simulink model "flare_mode"  (R2020b)
settings: Solver=VariableStepAuto  StartTime=0.0  StopTime=10.0  RelTol=1e-3
values from neighbouring files (symbols this model uses):
  Initial_elevator = -4.1    [Masterscript.m]
  Initial_throttle = 1000    [Masterscript.m]
  tau = 1.1233    [Masterscript.m]
  V_ref = 300    [Masterscript.m]
libraries: pid_lib x4, dspmathops x2
settings Model: Creator=niekv  LastModifiedBy=niekv

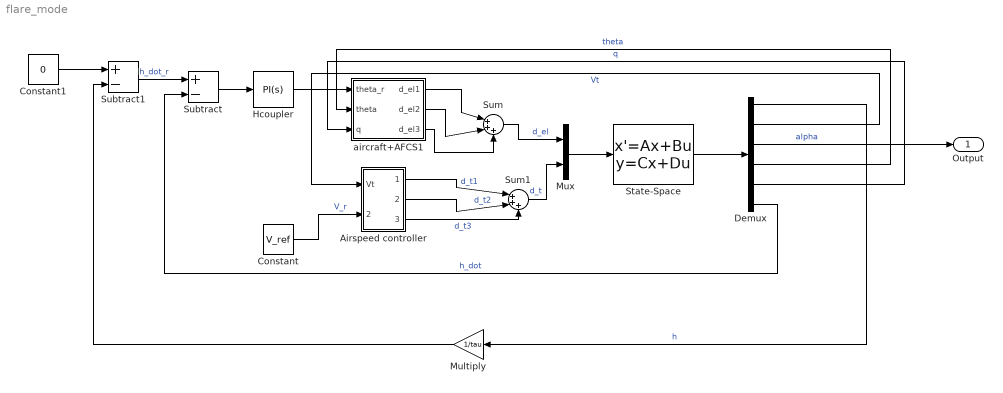
== system flare_mode ==
  Airspeed controller : Subsystem
  Constant : Constant  Value=V_ref
  Constant1 : Constant  Value=0
  Demux : Demux  Outputs=6
  Hcoupler : pid_lib/PID Controller  Controller=PI  Form=Parallel  TimeDomain=Continuous-time  UseExternalTs=off  SampleTime=-1  IntegratorMethod=Forward Euler  FilterMethod=Forward Euler  ControllerParametersSource=internal  P=1  I=0.1  D=0  UseFilter=on  N=100  TunerSelectOption=Transfer Function Based (PID Tuner App)  InitialConditionSource=internal  InitialConditionForIntegrator=0  InitialConditionForFilter=0  DifferentiatorICPrevScaledInput=0  ExternalReset=none  TrackingMode=off  Kt=1  LimitOutput=off  SatLimitsSource=internal  UpperSaturationLimit=inf  LowerSaturationLimit=-inf  LinearizeAsGain=on  AntiWindupMode=none  Kb=1  POutMin=[]  POutMax=[]  IOutMin=[]  IOutMax=[]  DOutMin=[]  DOutMax=[]  NOutMin=[]  NOutMax=[]  SumOutMin=[]  SumOutMax=[]  SaturationOutMin=[]  SaturationOutMax=[]  PParamMin=[]  PParamMax=[]  IParamMin=[]  IParamMax=[]  DParamMin=[]  DParamMax=[]  NParamMin=[]  NParamMax=[]  KbParamMin=[]  KbParamMax=[]  KtParamMin=[]  KtParamMax=[]  KbOutMin=[]  KbOutMax=[]  KtOutMin=[]  KtOutMax=[]  IntegratorOutMin=[]  IntegratorOutMax=[]  FilterOutMin=[]  FilterOutMax=[]  SumI1OutMin=[]  SumI1OutMax=[]  SumI2OutMin=[]  SumI2OutMax=[]  SumI3OutMin=[]  SumI3OutMax=[]  SumI4OutMin=[]  SumI4OutMax=[]  SumDOutMin=[]  SumDOutMax=[]  DifferentiatorOutMin=[]  DifferentiatorOutMax=[]  FilterDiffOutCoefMin=[]  FilterDiffOutCoefMax=[]  ReciprocalOutMin=[]  ReciprocalOutMax=[]  SumDenOutMin=[]  SumDenOutMax=[]  SumNumOutMin=[]  SumNumOutMax=[]  DivideOutMin=[]  DivideOutMax=[]  UdiffTsProdOutMin=[]  UdiffTsProdOutMax=[]  NTsProdOutMin=[]  NTsProdOutMax=[]  UintegralTsProdOutMin=[]  UintegralTsProdOutMax=[]  UngainTsProdOutMin=[]  UngainTsProdOutMax=[]  IntegratorContinuousStateAttributes=''  IntegratorStateMustResolveToSignalObject=off  IntegratorRTWStateStorageClass=Auto  FilterContinuousStateAttributes=''  FilterStateMustResolveToSignalObject=off  FilterRTWStateStorageClass=Auto  ParallelPVariant=InternalParameters  IdealPVariant=Disabled  IVariant=InternalParameters  DVariant=Disabled  IntegratorVariant=Continuous  SatVariant=Disabled  AWVariant=Passthrough  PCopyVariant=Disabled  TRVariant=Disabled  FdbkBlocksVariant=Forward  IdealPFdbkVariant=Disabled  SatFdbkVariant=Disabled  DerivativeFilterVariant=Disabled  NVariant=Disabled  NCopyVariant=Disabled_SignalSpec  FilterICVariant=Disabled  IntegratorICVariant=InternalICs  ExternalResetVariant=Disabled  TRSumVariant=Passthrough  SumFdbkVariant=Disabled  SumVariant=Sum_PI  TsampFilterVariant=InternalTs  TsampNgainVariant=Passthrough  TsampIntegralVariant=Passthrough  ExternalSaturationOutDataTypeStr=Inherit: Same as second input
  Multiply : Gain  Gain=1/tau
  Mux : Mux  Inputs=2
  State-Space : StateSpace  A=[0 0 -300 300 0; 0.0001317 -0.0291 2.13 -32.17 -2.895; 3.154e-06 -0.000697 -0.5447 4.55e-13 0.9152; 0 0 0 0 1; -4.699e-21 1.038e-18 0.3303 0 -0.8169]  B=[0 0; -0.004534 0.001544; -0.001116 -9.493e-07; 0 0 ; -0.05702 0]  C=[1 0 0 0 0; 0 1 0 0 0; 0 0 1 0 0; 0 0 0 1 0; 0 0 0 0 1; 0 0 -300 300 0]  D=[0 0; 0 0; 0 0; 0 0; 0 0; 0 0]  InitialCondition=[5000; 300; 10.4511; 10.4511; 0]  ContinuousStateAttributes={'h', 'Vt', 'alpha', 'theta', 'q'}
  Subtract : Sum  Inputs=+-
  Subtract1 : Sum  Inputs=+-
  Sum : Sum  Inputs=|+++
  Sum1 : Sum  Inputs=|+++
  aircraft+AFCS1 : Subsystem
  Output : Outport
  wires:
  State-Space/1 -> Demux/1
  Demux/2 -> Airspeed controller/1(Vt)  "Vt"
  Demux/3 -> Output/1  "alpha"
  Demux/4 -> aircraft+AFCS1/2(theta)  "theta"
  Demux/5 -> aircraft+AFCS1/3(q)  "q"
  Demux/6 -> Subtract/2  "h_dot"
  Mux/1 -> State-Space/1
  Sum1/1 -> Mux/2  "d_t"
  Sum/1 -> Mux/1  "d_el"
  Airspeed controller/3(d_t3) -> Sum1/3  "d_t3"
  Constant/1 -> Airspeed controller/2(V_r)  "V_r"
  Airspeed controller/2(d_t2) -> Sum1/2  "d_t2"
  Airspeed controller/1(d_t1) -> Sum1/1  "d_t1"
  aircraft+AFCS1/3(d_el3) -> Sum/3
  aircraft+AFCS1/2(d_el2) -> Sum/2
  aircraft+AFCS1/1(d_el1) -> Sum/1
  Hcoupler/1 -> aircraft+AFCS1/1(theta_r)
  Subtract/1 -> Hcoupler/1
  Demux/1 -> Multiply/1  "h"
  Subtract1/1 -> Subtract/1  "h_dot_r"
  Multiply/1 -> Subtract1/2
  Constant1/1 -> Subtract1/1

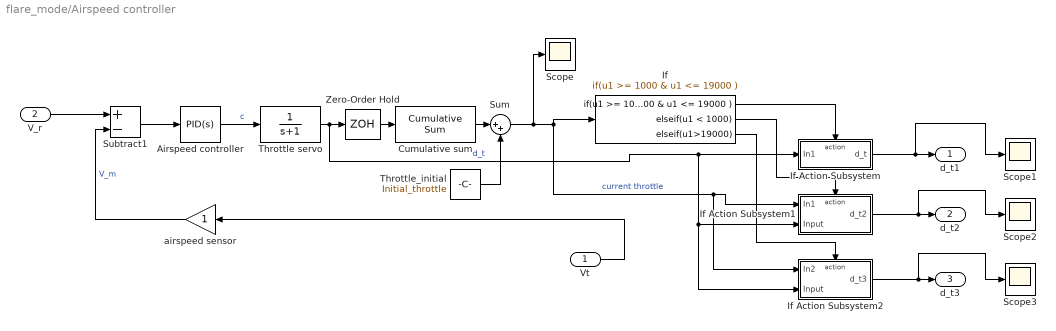
== system flare_mode/Airspeed controller ==
  Vt : Inport
  V_r : Inport  Port=2
  Airspeed controller : pid_lib/PID Controller  Controller=PID  Form=Parallel  TimeDomain=Continuous-time  UseExternalTs=off  SampleTime=-1  IntegratorMethod=Forward Euler  FilterMethod=Forward Euler  ControllerParametersSource=internal  P=1  I=0  D=0  UseFilter=on  N=100  TunerSelectOption=Transfer Function Based (PID Tuner App)  InitialConditionSource=internal  InitialConditionForIntegrator=0  InitialConditionForFilter=0  DifferentiatorICPrevScaledInput=0  ExternalReset=none  TrackingMode=off  Kt=1  LimitOutput=off  SatLimitsSource=internal  UpperSaturationLimit=inf  LowerSaturationLimit=-inf  LinearizeAsGain=on  AntiWindupMode=none  Kb=1  POutMin=[]  POutMax=[]  IOutMin=[]  IOutMax=[]  DOutMin=[]  DOutMax=[]  NOutMin=[]  NOutMax=[]  SumOutMin=[]  SumOutMax=[]  SaturationOutMin=[]  SaturationOutMax=[]  PParamMin=[]  PParamMax=[]  IParamMin=[]  IParamMax=[]  DParamMin=[]  DParamMax=[]  NParamMin=[]  NParamMax=[]  KbParamMin=[]  KbParamMax=[]  KtParamMin=[]  KtParamMax=[]  KbOutMin=[]  KbOutMax=[]  KtOutMin=[]  KtOutMax=[]  IntegratorOutMin=[]  IntegratorOutMax=[]  FilterOutMin=[]  FilterOutMax=[]  SumI1OutMin=[]  SumI1OutMax=[]  SumI2OutMin=[]  SumI2OutMax=[]  SumI3OutMin=[]  SumI3OutMax=[]  SumI4OutMin=[]  SumI4OutMax=[]  SumDOutMin=[]  SumDOutMax=[]  DifferentiatorOutMin=[]  DifferentiatorOutMax=[]  FilterDiffOutCoefMin=[]  FilterDiffOutCoefMax=[]  ReciprocalOutMin=[]  ReciprocalOutMax=[]  SumDenOutMin=[]  SumDenOutMax=[]  SumNumOutMin=[]  SumNumOutMax=[]  DivideOutMin=[]  DivideOutMax=[]  UdiffTsProdOutMin=[]  UdiffTsProdOutMax=[]  NTsProdOutMin=[]  NTsProdOutMax=[]  UintegralTsProdOutMin=[]  UintegralTsProdOutMax=[]  UngainTsProdOutMin=[]  UngainTsProdOutMax=[]  IntegratorContinuousStateAttributes=''  IntegratorStateMustResolveToSignalObject=off  IntegratorRTWStateStorageClass=Auto  FilterContinuousStateAttributes=''  FilterStateMustResolveToSignalObject=off  FilterRTWStateStorageClass=Auto  ParallelPVariant=InternalParameters  IdealPVariant=Disabled  IVariant=InternalParameters  DVariant=InternalParameters  IntegratorVariant=Continuous  SatVariant=Disabled  AWVariant=Passthrough  PCopyVariant=Disabled  TRVariant=Disabled  FdbkBlocksVariant=Forward  IdealPFdbkVariant=Disabled  SatFdbkVariant=Disabled  DerivativeFilterVariant=ContFilter  NVariant=InternalParameters  NCopyVariant=Disabled  FilterICVariant=InternalICsFilter  IntegratorICVariant=InternalICs  ExternalResetVariant=Disabled  TRSumVariant=Passthrough  SumFdbkVariant=Disabled  SumVariant=Sum_PID  TsampFilterVariant=InternalTs  TsampNgainVariant=Passthrough  TsampIntegralVariant=Passthrough  ExternalSaturationOutDataTypeStr=Inherit: Same as second input
  Cumulative sum : dspmathops/Cumulative Sum  dim=Channels (running sum)  InputProcessing=Columns as channels (frame based)  reset_popup=None  roundingMode=Floor  overflowMode=off  outputDataTypeStr=Inherit: Same as accumulator  outputMin=[]  outputMax=[]  outputLastDataTypeStr=Inherit: Same as accumulator
  If : If  IfExpression=u1 >= 1000 & u1 <= 19000  ElseIfExpressions=u1 < 1000, u1>19000  ShowElse=off
  If Action Subsystem : Subsystem  TreatAsAtomicUnit=on
  If Action Subsystem1 : Subsystem  TreatAsAtomicUnit=on
  If Action Subsystem2 : Subsystem  TreatAsAtomicUnit=on
  Scope{,1..3} (4 alike) : Scope
  Subtract1 : Sum  Inputs=+-
  Sum : Sum  Inputs=|++
  Throttle servo : TransferFcn  Denominator=[1 1]
  Throttle_initial : Constant  Value=Initial_throttle
  Zero-Order Hold : ZeroOrderHold  SampleTime=0.1
  airspeed sensor : Gain
  d_t1 : Outport
  d_t2 : Outport  Port=2
  d_t3 : Outport  Port=3
  wires:
  Subtract1/1 -> Airspeed controller/1
  airspeed sensor/1 -> Subtract1/2  "V_m"
  Throttle servo/1 -> Zero-Order Hold/1, If Action Subsystem2/2(Input), If Action Subsystem1/2(Input), If Action Subsystem/1(In1)  "d_t"
  V_r/1 -> Subtract1/1
  Airspeed controller/1 -> Throttle servo/1  "c"
  Vt/1 -> airspeed sensor/1
  Throttle_initial/1 -> Sum/2
  Cumulative sum/1 -> Sum/1
  Sum/1 -> Scope/1, If Action Subsystem2/1(In2), If Action Subsystem1/1(In1), If/1  "current throttle"
  If/1 -> If Action Subsystem/Action
  If Action Subsystem/1(d_t) -> Scope1/1, d_t1/1
  If/2 -> If Action Subsystem1/Action
  If/3 -> If Action Subsystem2/Action
  If Action Subsystem2/1(d_t3) -> Scope3/1, d_t3/1
  If Action Subsystem1/1(d_t2) -> Scope2/1, d_t2/1
  Zero-Order Hold/1 -> Cumulative sum/1

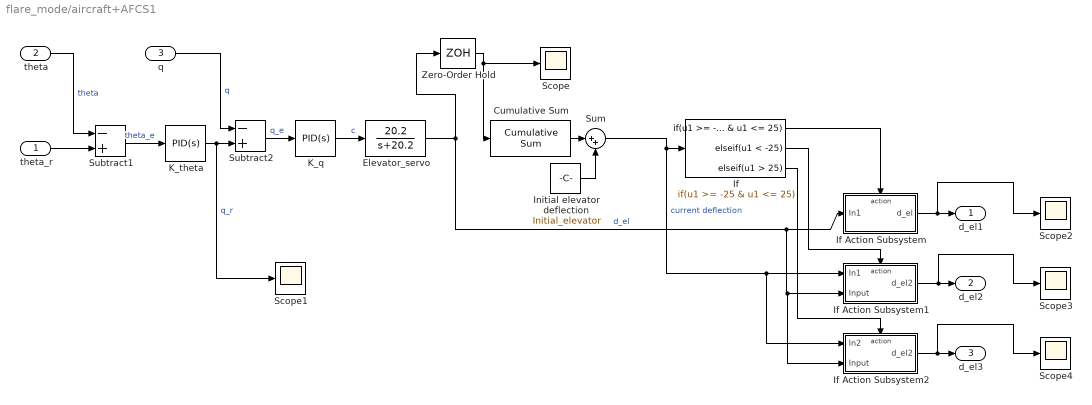
== system flare_mode/aircraft+AFCS1 ==
  theta_r : Inport
  theta : Inport  Port=2
  q : Inport  Port=3
  Cumulative Sum : dspmathops/Cumulative Sum  dim=Channels (running sum)  InputProcessing=Columns as channels (frame based)  reset_popup=None  roundingMode=Floor  overflowMode=off  outputDataTypeStr=Inherit: Same as accumulator  outputMin=[]  outputMax=[]  outputLastDataTypeStr=Inherit: Same as accumulator
  Elevator_servo : TransferFcn  Numerator=[20.2]  Denominator=[1 20.2]  ContinuousStateAttributes='elevator_servo'
  If : If  IfExpression=u1 >= -25 & u1 <= 25  ElseIfExpressions=u1 < -25, u1 > 25  ShowElse=off
  If Action Subsystem : Subsystem  TreatAsAtomicUnit=on
  If Action Subsystem1 : Subsystem  TreatAsAtomicUnit=on
  If Action Subsystem2 : Subsystem  TreatAsAtomicUnit=on
  Initial elevator deflection : Constant  Value=Initial_elevator
  K_q : pid_lib/PID Controller  Controller=PID  Form=Parallel  TimeDomain=Continuous-time  UseExternalTs=off  SampleTime=-1  IntegratorMethod=Forward Euler  FilterMethod=Forward Euler  ControllerParametersSource=internal  P=1  I=0  D=0  UseFilter=on  N=100  TunerSelectOption=Transfer Function Based (PID Tuner App)  InitialConditionSource=internal  InitialConditionForIntegrator=0  InitialConditionForFilter=0  DifferentiatorICPrevScaledInput=0  ExternalReset=none  TrackingMode=off  Kt=1  LimitOutput=off  SatLimitsSource=internal  UpperSaturationLimit=inf  LowerSaturationLimit=-inf  LinearizeAsGain=on  AntiWindupMode=none  Kb=1  POutMin=[]  POutMax=[]  IOutMin=[]  IOutMax=[]  DOutMin=[]  DOutMax=[]  NOutMin=[]  NOutMax=[]  SumOutMin=[]  SumOutMax=[]  SaturationOutMin=[]  SaturationOutMax=[]  PParamMin=[]  PParamMax=[]  IParamMin=[]  IParamMax=[]  DParamMin=[]  DParamMax=[]  NParamMin=[]  NParamMax=[]  KbParamMin=[]  KbParamMax=[]  KtParamMin=[]  KtParamMax=[]  KbOutMin=[]  KbOutMax=[]  KtOutMin=[]  KtOutMax=[]  IntegratorOutMin=[]  IntegratorOutMax=[]  FilterOutMin=[]  FilterOutMax=[]  SumI1OutMin=[]  SumI1OutMax=[]  SumI2OutMin=[]  SumI2OutMax=[]  SumI3OutMin=[]  SumI3OutMax=[]  SumI4OutMin=[]  SumI4OutMax=[]  SumDOutMin=[]  SumDOutMax=[]  DifferentiatorOutMin=[]  DifferentiatorOutMax=[]  FilterDiffOutCoefMin=[]  FilterDiffOutCoefMax=[]  ReciprocalOutMin=[]  ReciprocalOutMax=[]  SumDenOutMin=[]  SumDenOutMax=[]  SumNumOutMin=[]  SumNumOutMax=[]  DivideOutMin=[]  DivideOutMax=[]  UdiffTsProdOutMin=[]  UdiffTsProdOutMax=[]  NTsProdOutMin=[]  NTsProdOutMax=[]  UintegralTsProdOutMin=[]  UintegralTsProdOutMax=[]  UngainTsProdOutMin=[]  UngainTsProdOutMax=[]  IntegratorContinuousStateAttributes=''  IntegratorStateMustResolveToSignalObject=off  IntegratorRTWStateStorageClass=Auto  FilterContinuousStateAttributes=''  FilterStateMustResolveToSignalObject=off  FilterRTWStateStorageClass=Auto  ParallelPVariant=InternalParameters  IdealPVariant=Disabled  IVariant=InternalParameters  DVariant=InternalParameters  IntegratorVariant=Continuous  SatVariant=Disabled  AWVariant=Passthrough  PCopyVariant=Disabled  TRVariant=Disabled  FdbkBlocksVariant=Forward  IdealPFdbkVariant=Disabled  SatFdbkVariant=Disabled  DerivativeFilterVariant=ContFilter  NVariant=InternalParameters  NCopyVariant=Disabled  FilterICVariant=InternalICsFilter  IntegratorICVariant=InternalICs  ExternalResetVariant=Disabled  TRSumVariant=Passthrough  SumFdbkVariant=Disabled  SumVariant=Sum_PID  TsampFilterVariant=InternalTs  TsampNgainVariant=Passthrough  TsampIntegralVariant=Passthrough  ExternalSaturationOutDataTypeStr=Inherit: Same as second input
  K_theta : pid_lib/PID Controller  Controller=PID  Form=Parallel  TimeDomain=Continuous-time  UseExternalTs=off  SampleTime=-1  IntegratorMethod=Forward Euler  FilterMethod=Forward Euler  ControllerParametersSource=internal  P=1  I=0  D=0  UseFilter=on  N=100  TunerSelectOption=Transfer Function Based (PID Tuner App)  InitialConditionSource=internal  InitialConditionForIntegrator=0  InitialConditionForFilter=0  DifferentiatorICPrevScaledInput=0  ExternalReset=none  TrackingMode=off  Kt=1  LimitOutput=off  SatLimitsSource=internal  UpperSaturationLimit=inf  LowerSaturationLimit=-inf  LinearizeAsGain=on  AntiWindupMode=none  Kb=1  POutMin=[]  POutMax=[]  IOutMin=[]  IOutMax=[]  DOutMin=[]  DOutMax=[]  NOutMin=[]  NOutMax=[]  SumOutMin=[]  SumOutMax=[]  SaturationOutMin=[]  SaturationOutMax=[]  PParamMin=[]  PParamMax=[]  IParamMin=[]  IParamMax=[]  DParamMin=[]  DParamMax=[]  NParamMin=[]  NParamMax=[]  KbParamMin=[]  KbParamMax=[]  KtParamMin=[]  KtParamMax=[]  KbOutMin=[]  KbOutMax=[]  KtOutMin=[]  KtOutMax=[]  IntegratorOutMin=[]  IntegratorOutMax=[]  FilterOutMin=[]  FilterOutMax=[]  SumI1OutMin=[]  SumI1OutMax=[]  SumI2OutMin=[]  SumI2OutMax=[]  SumI3OutMin=[]  SumI3OutMax=[]  SumI4OutMin=[]  SumI4OutMax=[]  SumDOutMin=[]  SumDOutMax=[]  DifferentiatorOutMin=[]  DifferentiatorOutMax=[]  FilterDiffOutCoefMin=[]  FilterDiffOutCoefMax=[]  ReciprocalOutMin=[]  ReciprocalOutMax=[]  SumDenOutMin=[]  SumDenOutMax=[]  SumNumOutMin=[]  SumNumOutMax=[]  DivideOutMin=[]  DivideOutMax=[]  UdiffTsProdOutMin=[]  UdiffTsProdOutMax=[]  NTsProdOutMin=[]  NTsProdOutMax=[]  UintegralTsProdOutMin=[]  UintegralTsProdOutMax=[]  UngainTsProdOutMin=[]  UngainTsProdOutMax=[]  IntegratorContinuousStateAttributes=''  IntegratorStateMustResolveToSignalObject=off  IntegratorRTWStateStorageClass=Auto  FilterContinuousStateAttributes=''  FilterStateMustResolveToSignalObject=off  FilterRTWStateStorageClass=Auto  ParallelPVariant=InternalParameters  IdealPVariant=Disabled  IVariant=InternalParameters  DVariant=InternalParameters  IntegratorVariant=Continuous  SatVariant=Disabled  AWVariant=Passthrough  PCopyVariant=Disabled  TRVariant=Disabled  FdbkBlocksVariant=Forward  IdealPFdbkVariant=Disabled  SatFdbkVariant=Disabled  DerivativeFilterVariant=ContFilter  NVariant=InternalParameters  NCopyVariant=Disabled  FilterICVariant=InternalICsFilter  IntegratorICVariant=InternalICs  ExternalResetVariant=Disabled  TRSumVariant=Passthrough  SumFdbkVariant=Disabled  SumVariant=Sum_PID  TsampFilterVariant=InternalTs  TsampNgainVariant=Passthrough  TsampIntegralVariant=Passthrough  ExternalSaturationOutDataTypeStr=Inherit: Same as second input
  Scope{,1..4} (5 alike) : Scope
  Subtract1 : Sum  Inputs=-+
  Subtract2 : Sum  Inputs=-+
  Sum : Sum  Inputs=|++
  Zero-Order Hold : ZeroOrderHold  SampleTime=0.1
  d_el1 : Outport
  d_el2 : Outport  Port=2
  d_el3 : Outport  Port=3
  wires:
  Subtract2/1 -> K_q/1  "q_e"
  K_theta/1 -> Scope1/1, Subtract2/2  "q_r"
  theta_r/1 -> Subtract1/2
  theta/1 -> Subtract1/1  "theta"
  K_q/1 -> Elevator_servo/1  "c"
  q/1 -> Subtract2/1  "q"
  Subtract1/1 -> K_theta/1  "theta_e"
  Elevator_servo/1 -> Zero-Order Hold/1, If Action Subsystem2/2(Input), If Action Subsystem1/2(Input), If Action Subsystem/1(In1)  "d_el"
  Initial elevator deflection/1 -> Sum/2
  Cumulative Sum/1 -> Sum/1
  Sum/1 -> If Action Subsystem2/1(In2), If Action Subsystem1/1(In1), If/1  "current deflection"
  If/1 -> If Action Subsystem/Action
  If Action Subsystem/1(d_el) -> Scope2/1, d_el1/1
  If/2 -> If Action Subsystem1/Action
  If Action Subsystem1/1(d_el2) -> Scope3/1, d_el2/1
  If/3 -> If Action Subsystem2/Action
  If Action Subsystem2/1(d_el2) -> Scope4/1, d_el3/1
  Zero-Order Hold/1 -> Cumulative Sum/1, Scope/1

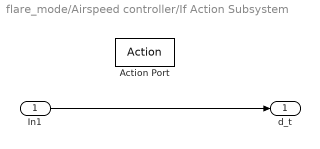
== system flare_mode/Airspeed controller/If Action Subsystem ==
  In1 : Inport
  Action Port : ActionPort
  d_t : Outport
  wires:
  In1/1 -> d_t/1

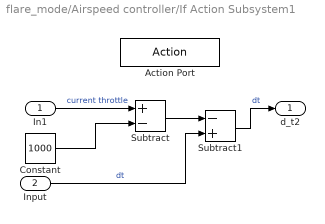
== system flare_mode/Airspeed controller/If Action Subsystem1 ==
  In1 : Inport
  Input : Inport  Port=2
  Action Port : ActionPort
  Constant : Constant  Value=1000
  Subtract : Sum  Inputs=+-
  Subtract1 : Sum  Inputs=-+
  d_t2 : Outport
  wires:
  In1/1 -> Subtract/1  "current throttle"
  Input/1 -> Subtract1/2  "dt"
  Constant/1 -> Subtract/2
  Subtract/1 -> Subtract1/1
  Subtract1/1 -> d_t2/1  "dt"

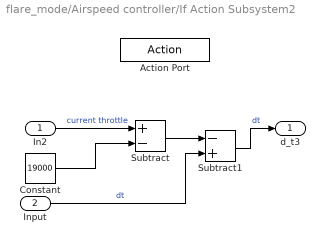
== system flare_mode/Airspeed controller/If Action Subsystem2 ==
  In2 : Inport
  Input : Inport  Port=2
  Action Port : ActionPort
  Constant : Constant  Value=19000
  Subtract : Sum  Inputs=+-
  Subtract1 : Sum  Inputs=-+
  d_t3 : Outport
  wires:
  Subtract1/1 -> d_t3/1  "dt"
  Input/1 -> Subtract1/2  "dt"
  Constant/1 -> Subtract/2
  Subtract/1 -> Subtract1/1
  In2/1 -> Subtract/1  "current throttle"

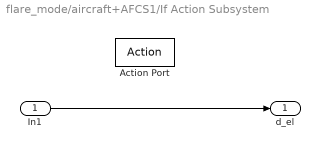
== system flare_mode/aircraft+AFCS1/If Action Subsystem ==
  In1 : Inport
  Action Port : ActionPort
  d_el : Outport
  wires:
  In1/1 -> d_el/1

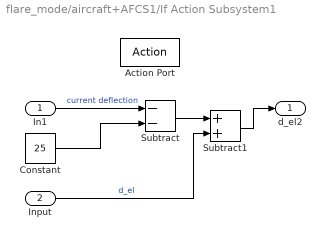
== system flare_mode/aircraft+AFCS1/If Action Subsystem1 ==
  In1 : Inport
  Input : Inport  Port=2
  Action Port : ActionPort
  Constant : Constant  Value=25
  Subtract : Sum  Inputs=--
  Subtract1 : Sum
  d_el2 : Outport
  wires:
  In1/1 -> Subtract/1  "current deflection"
  Constant/1 -> Subtract/2
  Subtract/1 -> Subtract1/1
  Input/1 -> Subtract1/2  "d_el"
  Subtract1/1 -> d_el2/1

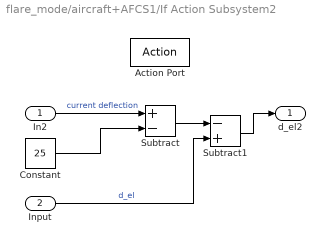
== system flare_mode/aircraft+AFCS1/If Action Subsystem2 ==
  In2 : Inport
  Input : Inport  Port=2
  Action Port : ActionPort
  Constant : Constant  Value=25
  Subtract : Sum  Inputs=+-
  Subtract1 : Sum  Inputs=-+
  d_el2 : Outport
  wires:
  Subtract1/1 -> d_el2/1
  Input/1 -> Subtract1/2  "d_el"
  In2/1 -> Subtract/1  "current deflection"
  Constant/1 -> Subtract/2
  Subtract/1 -> Subtract1/1
